simulink model "lookup_nD_TestGen13"  (R2017b)
settings: Solver=FixedStepDiscrete  StartTime=0.0  StopTime=10.0  RelTol=1e-3
settings Model: Creator=ktrinh  LastModifiedBy=ktrinh
settings DebuggingCC: ParameterOverflowMsg=none

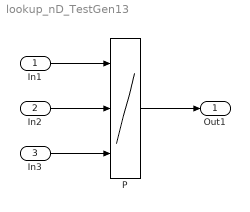
== system lookup_nD_TestGen13 ==
  In1 : Inport  OutMin=0  OutMax=127  OutDataTypeStr=uint32  PortDimensions=[2,3]
  In2 : Inport  Port=2  OutMin=0  OutMax=127  OutDataTypeStr=uint32
  In3 : Inport  Port=3  OutMin=0  OutMax=127  OutDataTypeStr=uint32
  P : Lookup_n-D  NumberOfTableDimensions=3  BreakpointsForDimension1=[9.46335518355963;78.6151632013826]  BreakpointsForDimension2=[50.9512991669223;61.2059107136011;80.98513048821;83.1699707454656;86.4479007969709]  BreakpointsForDimension3=[13.465737608242;60.0302613265942;82.0980658586859]  BreakpointsForDimension1DataTypeStr=single  BreakpointsForDimension2DataTypeStr=single  BreakpointsForDimension3DataTypeStr=single  Table=reshape(repmat([4 5 6 7 8;16 19 20 21 22;10 18 23 24 25],1,2),[2,5,3])  InterpMethod=Flat  ExtrapMethod=Clip  InternalRulePriority=Speed  OutDataTypeStr=single  RndMeth=Zero  SaturateOnIntegerOverflow=on  InputSameDT=on
  Out1 : Outport
  wires:
  In1/1 -> P/1
  In2/1 -> P/2
  In3/1 -> P/3
  P/1 -> Out1/1
